simulink library "Lib_Cntrl_CorrectedSpeed_TMATS"  (R2012b)
settings: Solver=ode45  StartTime=0.0  StopTime=10.0  RelTol=1e-3
Description:
  | Thomas Modules
settings Model: Creator=jwchapm2  LastModifiedBy=jwchapm2

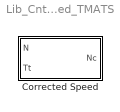
== system Lib_Cntrl_CorrectedSpeed_TMATS ==
  Corrected Speed : Subsystem  mask(T-MATS: Corrected Speed Library Block){C_TSTD_M=518.67}
      mask prompts: C_TSTD_M "C_TSTD_M - Standard Day Temperature [degR]"
      mask help:
      | This block calculates corrected speed.
      | Nc = N / sqrt(theta)
      mask Help: web(which('Control_TMATS_CS.html'),'-helpbrowser')

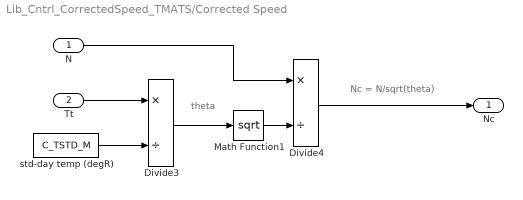
== system Lib_Cntrl_CorrectedSpeed_TMATS/Corrected Speed ==
  note: Nc = N/sqrt(theta)
  note: theta
  N : Inport
  Tt : Inport  Port=2
  Divide3 : Product  Inputs=*/
  Divide4 : Product  Inputs=*/
  Math Function1 : Math  Operator=sqrt  SaturateOnIntegerOverflow=on
  std-day temp (degR) : Constant  Value=C_TSTD_M
  Nc : Outport
  wires:
  Divide4/1 -> Nc/1
  N/1 -> Divide4/1
  Math Function1/1 -> Divide4/2
  Divide3/1 -> Math Function1/1
  std-day temp (degR)/1 -> Divide3/2
  Tt/1 -> Divide3/1
